simulink model "HighLevelLowLevel_SITLA 2"  (R2023b)
settings: Solver=FixedStepAuto  StartTime=0.0  StopTime=100  FixedStep=0.0025  RelTol=1e-3
InitFcn:
  | startup
model workspace (MAT data in the model file):
  Cd = 2.24197803e-06
  Ct = 0.00010297
  Ixx = 113600
  Iyy = 113600
  Izz = 22620
  h = 0.05
values from neighbouring files (symbols this model uses):
  g = 9.806    [startup.m]
  I = [0.42 0 0; 0 0.42 0; 0 0 0.642]    [startup.m]
  l = 0.053336    [startup.m]
  m = 7.4    [startup.m]
  sample_rate = 0.0025    [startup.m]
libraries: simulink_extras x12, matrix_library x9, AP_Conector0x2810x29 x2, aerolibanimutils x1, shared6dof x1, commchan3 x1
settings Model: Creator=awahm  LastModifiedBy=okmatteson
settings OptimizationCC: DefaultParameterBehavior=Inlined  UseDivisionForNetSlopeComputation=on  GainParamInheritBuiltInType=on  UseFloatMulNetSlope=on  OptimizeBlockIOStorage=off  ZeroExternalMemoryAtStartup=off  ZeroInternalMemoryAtStartup=off  LifeSpan=1  OptimizeDataStoreBuffers=off  BusAssignmentInplaceUpdate=off
settings DebuggingCC: SFUnexpectedBacktrackingDiag=warning  SFNoUnconditionalDefaultTransitionDiag=warning
settings RTWCC: GenerateReport=on  BuildConfiguration=Debug  LaunchReport=on  TargetLang=C++
settings CodeAppCC: ForceParamTrailComments=on  MATLABSourceComments=on  EnableCustomComments=on
settings GRTTargetCC: TargetLangStandard=C++11 (ISO)  CombineSignalStateStructs=on  CodeInterfacePackaging=C++ class  SupportVariableSizeSignals=on  MultiInstanceErrorCode=Warning

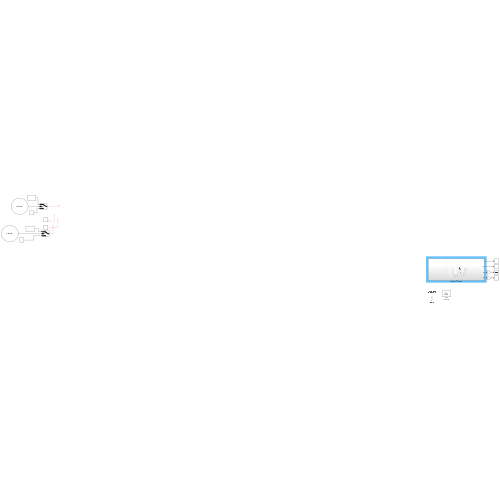
[thumbnail: Simulink's stored preview of the top-level diagram]
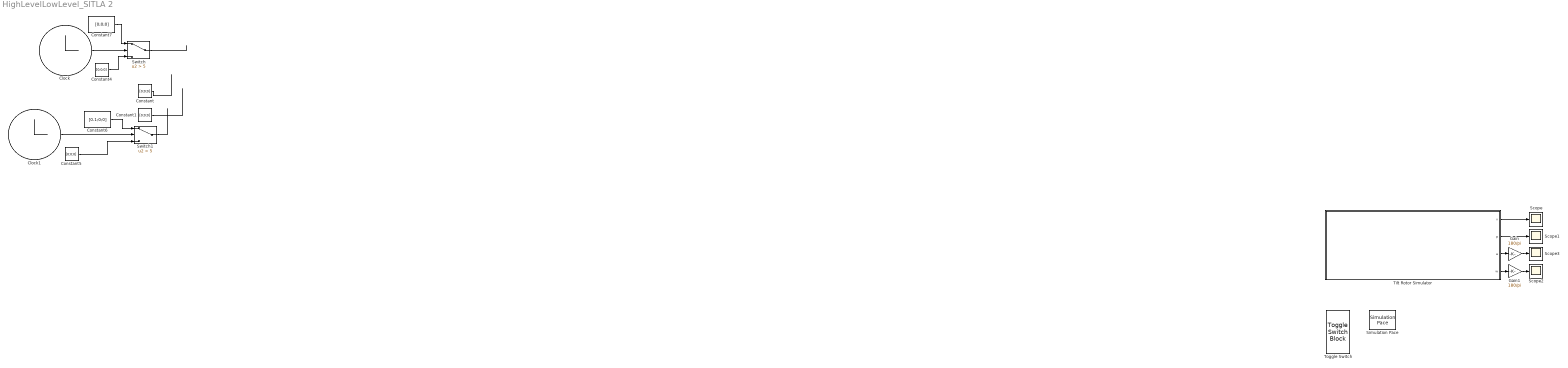
== system HighLevelLowLevel_SITLA 2 ==
  Clock : Clock
  Clock1 : Clock
  Constant{,1,4..5,7} (5 alike) : Constant  Value=[0;0;0]
  Constant6 : Constant  Value=[0.1;0;0]
  Gain : Gain  Gain=180/pi
  Gain1 : Gain  Gain=180/pi
  Scope{,1..3} (4 alike) : Scope
  Simulation Pace : aerolibanimutils/Simulation Pace  SimulationPace=1  SleepMode=Auto  OutputPaceError=off  SampleTime=sample_rate
  Switch : Switch  Criteria=u2 > Threshold  Threshold=5  SaturateOnIntegerOverflow=off  InputSameDT=off
  Switch1 : Switch  Criteria=u2 > Threshold  Threshold=5  SaturateOnIntegerOverflow=off  InputSameDT=off
  Tilt Rotor Simulator : Subsystem
  Toggle Switch : ToggleSwitchBlock
      settings: Values={{'Manual', 'Autonomous'}, [0 1]}
  wires:
  Constant/1 -> ?
  Switch1/1 -> ?
  Constant1/1 -> ?
  Clock/1 -> Switch/2
  Constant7/1 -> Switch/1
  Switch/1 -> ?
  Constant4/1 -> Switch/3
  Clock1/1 -> Switch1/2
  Constant6/1 -> Switch1/1
  Constant5/1 -> Switch1/3
  Tilt Rotor Simulator/1(v) -> Scope/1
  Tilt Rotor Simulator/4(w) -> Gain1/1
  Tilt Rotor Simulator/3(a) -> Gain/1
  Tilt Rotor Simulator/2(p) -> Scope1/1
  Gain/1 -> Scope3/1
  Gain1/1 -> Scope2/1

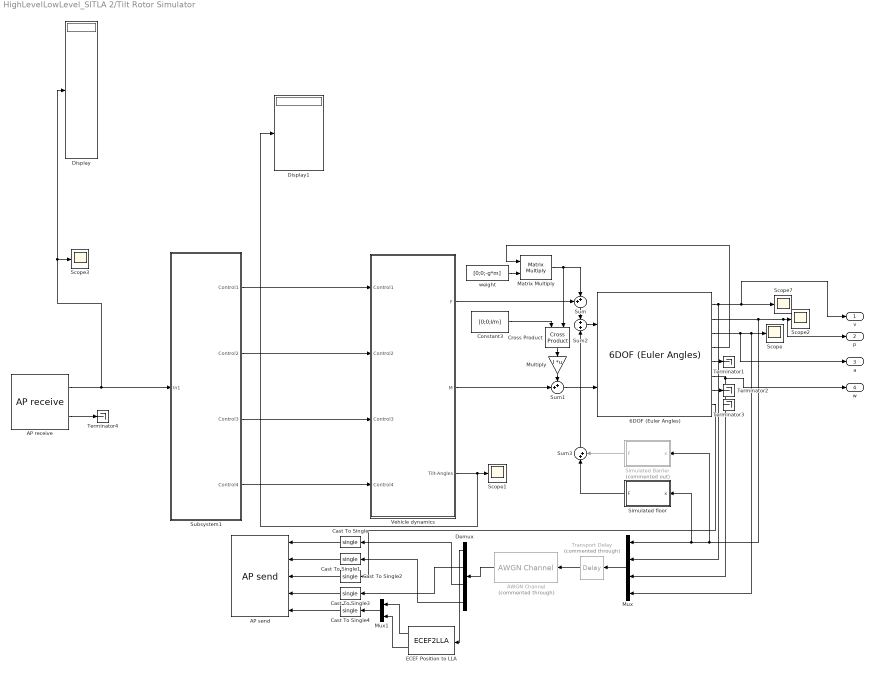
== system HighLevelLowLevel_SITLA 2/Tilt Rotor Simulator ==
  6DOF (Euler Angles) : shared6dof/6DOF (Euler Angles)  units=Metric (MKS)  mtype=Fixed  rep=Euler Angles  xme_0=[0 0 0]  Vm_0=[0 0 0]  eul_0=[0 0 0]  pm_0=[0 0 0]  mass_0=7.4  mass_e=0.5  mass_f=2.0  inertia=I  inertia_e=eye(3)  inertia_f=2*eye(3)  k_quat=1.0  vre_flag=on  abi_flag=off  aMode=0  xme_statename=''  Vm_statename=''  eul_statename=''  quat_statename=''  pm_statename=''  mass_statename=''
  AP receive : AP_Conector0x2810x29/AP receive  SystemSampleTime=-1  VariantActivationTime=update diagram  AllowFlexibleInterface=on  Latency=0  AutoFrameSizeCalculation=off
  AP send : AP_Conector0x2810x29/AP send  SystemSampleTime=-1  VariantActivationTime=update diagram  AllowFlexibleInterface=on  Latency=0  AutoFrameSizeCalculation=off
  AWGN Channel : commchan3/AWGN Channel  Commented=through  LegacyMode=on  NoiseMethod="Signal to noise ratio  (SNR)"  noiseMode="Signal to noise ratio  (SNR)"  EbNo=10  EsNo=10  SNR=10  BitsPerSymbol=1  SignalPower=1  SamplesPerSymbol=1  SymbolPeriod=1  VarianceSource=Parameter  Variance=1  RandomStream=Global stream  Seed=67  SimulateUsing=Code generation
  Cast To Single{,1..4} (5 alike) : DataTypeConversion  OutDataTypeStr=single  SaturateOnIntegerOverflow=off  RndMeth=Floor
  Constant3 : Constant  Value=[0;0;l/m]
  Cross Product : matrix_library/Cross Product
  Demux : Demux
  Display : Display
  Display1 : Display
  ECEF Position to LLA : ECEF2LLA
  Matrix Multiply : Product  Multiplication=Matrix(*)
  Multiply : Gain  Gain=I  Multiplication=Matrix(K*u)
  Mux : Mux
  Mux1 : Mux  Inputs=2
  Scope{,1..3,7} (5 alike) : Scope
  Simulated Barrier : MATLAB Function  Commented=on  TreatAsAtomicUnit=on  mask{x1=[0; -5], x2=[0; 5], E=1000000, thickness=0.1, A=0.5^2}
  Simulated floor : MATLAB Function  TreatAsAtomicUnit=on  mask{x1=[-100; -0.1], x2=[100; -0.1], E=1000000, thickness=0.1, A=0.5^2}
  Subsystem1 : Subsystem
  Sum : Sum  Inputs=++|
  Sum1 : Sum  Inputs=++|
  Sum2 : Sum  Inputs=+|+
  Sum3 : Sum  Inputs=|++
  Terminator{1..4} (4 alike) : Terminator
  Transport Delay : TransportDelay  Commented=through  DelayTime=0.006
  Vehicle dynamics : Subsystem
  weight : Constant  Value=[0;0;-g*m]
  v : Outport
  p : Outport  Port=2
  a : Outport  Port=3
  w : Outport  Port=4
  wires:
  6DOF (Euler Angles)/2 -> p/1, Scope2/1, Simulated Barrier/1(x), Simulated floor/1(x), Mux/1
  Mux/1 -> Transport Delay/1
  6DOF (Euler Angles)/6 -> w/1, Mux/3
  weight/1 -> Matrix Multiply/2
  Matrix Multiply/1 -> Cross Product/2, Sum/2
  Vehicle dynamics/1(F) -> Sum/1
  6DOF (Euler Angles)/8 -> Cast To Single2/1
  Vehicle dynamics/3(Tilt-Angles) -> Display1/1, Scope1/1
  Sum1/1 -> 6DOF (Euler Angles)/2
  AWGN Channel/1 -> Demux/1
  6DOF (Euler Angles)/1 -> v/1, Scope7/1, Mux/2
  Cross Product/1 -> Multiply/1
  Vehicle dynamics/2(M) -> Sum1/2
  6DOF (Euler Angles)/3 -> a/1, Mux/4, Scope/1
  6DOF (Euler Angles)/7 -> Terminator2/1
  Transport Delay/1 -> AWGN Channel/1
  6DOF (Euler Angles)/4 -> Matrix Multiply/1
  Constant3/1 -> Cross Product/1
  Multiply/1 -> Sum1/1
  6DOF (Euler Angles)/5 -> Terminator1/1
  Sum/1 -> Sum2/1
  Sum2/1 -> 6DOF (Euler Angles)/1
  Simulated Barrier/1(F) -> Sum3/2
  AP receive/2 -> Terminator4/1
  AP receive/1 -> Scope3/1, Display/1, Subsystem1/1(In1)
  Demux/1 -> ECEF Position to LLA/1
  Demux/2 -> Cast To Single3/1
  Demux/4 -> Cast To Single1/1
  Demux/3 -> Cast To Single/1
  Cast To Single/1 -> AP send/1
  Cast To Single1/1 -> AP send/2
  Cast To Single4/1 -> AP send/5
  Subsystem1/1(Control1) -> Vehicle dynamics/1(Control1)
  Subsystem1/2(Control2) -> Vehicle dynamics/2(Control2)
  Subsystem1/3(Control3) -> Vehicle dynamics/3(Control3)
  Subsystem1/4(Control4) -> Vehicle dynamics/4(Control4)
  ECEF Position to LLA/1 -> Mux1/1
  ECEF Position to LLA/2 -> Mux1/2
  Mux1/1 -> Cast To Single4/1
  Cast To Single3/1 -> AP send/4
  Cast To Single2/1 -> AP send/3
  Simulated floor/1(F) -> Sum3/1
  Sum3/1 -> Sum2/2

== system HighLevelLowLevel_SITLA 2/Tilt Rotor Simulator/Subsystem1 ==
  In1 : Inport
  Demux1 : Demux  Outputs=16
  Mux{,1..3} (4 alike) : Mux  Inputs=3
  Scope : Scope
  Scope1 : Scope
  Subsystem : Subsystem
  Control1 : Outport
  Control2 : Outport  Port=2
  Control3 : Outport  Port=3
  Control4 : Outport  Port=4
  wires:
  Demux1/1 -> Subsystem/1(In1)
  Demux1/2 -> Subsystem/2(In2)
  Demux1/3 -> Subsystem/3(In3)
  Demux1/4 -> Subsystem/4(In4)
  Demux1/5 -> Scope1/1, Subsystem/5(In5)
  Demux1/6 -> Subsystem/6(In6)
  Demux1/8 -> Subsystem/8(In8)
  Demux1/7 -> Subsystem/7(In7)
  Demux1/9 -> Subsystem/9(In9)
  Demux1/10 -> Subsystem/10(In10)
  Demux1/11 -> Subsystem/11(In11)
  Demux1/12 -> Subsystem/12(In12)
  In1/1 -> Demux1/1
  Subsystem/1(Out1) -> Mux/3
  Subsystem/5(Out5) -> Mux/2, Scope/1
  Subsystem/9(Out9) -> Mux/1
  Mux/1 -> Control1/1
  Mux1/1 -> Control2/1
  Subsystem/2(Out2) -> Mux1/3
  Subsystem/6(Out6) -> Mux1/2
  Subsystem/10(Out10) -> Mux1/1
  Mux2/1 -> Control3/1
  Subsystem/7(Out7) -> Mux2/2
  Subsystem/3(Out3) -> Mux2/3
  Subsystem/11(Out11) -> Mux2/1
  Mux3/1 -> Control4/1
  Subsystem/4(Out4) -> Mux3/3
  Subsystem/8(Out8) -> Mux3/2
  Subsystem/12(Out12) -> Mux3/1

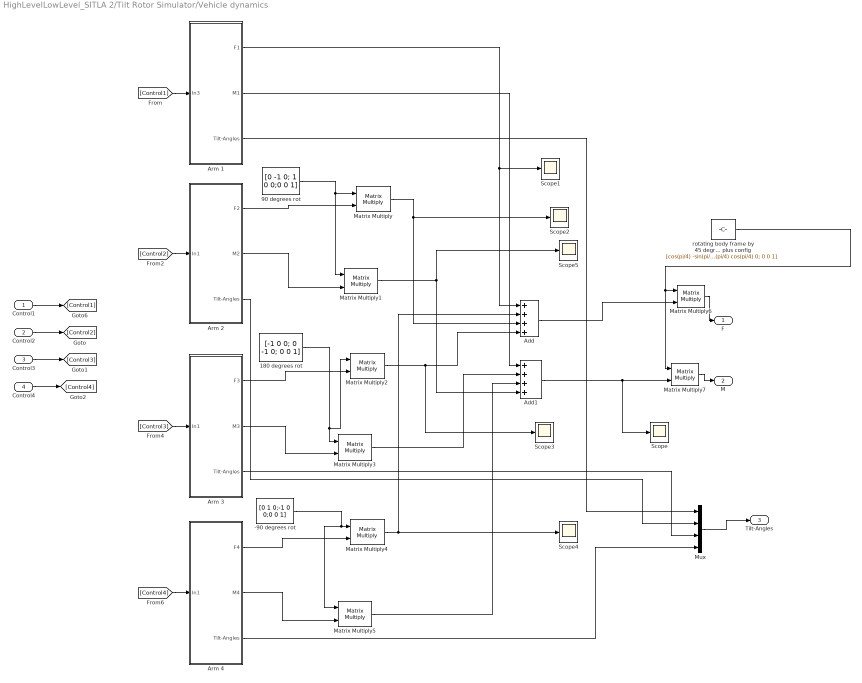
== system HighLevelLowLevel_SITLA 2/Tilt Rotor Simulator/Vehicle dynamics ==
  Control1 : Inport
  Control2 : Inport  Port=2
  Control3 : Inport  Port=3
  Control4 : Inport  Port=4
  -90 degrees rot : Constant  Value=[0 1 0;-1 0 0;0 0 1]
  180 degrees rot : Constant  Value=[-1 0 0; 0 -1 0; 0 0 1]
  90 degrees rot : Constant  Value=[0 -1 0; 1 0 0;0 0 1]
  Add : Sum  Inputs=++++
  Add1 : Sum  Inputs=++++
  Arm 1 : Subsystem
  Arm 2 : Subsystem
  Arm 3 : Subsystem
  Arm 4 : Subsystem
  Matrix Multiply{,1..7} (8 alike) : Product  Multiplication=Matrix(*)
  Mux : Mux
  Scope{,1..5} (6 alike) : Scope
  rotating body frame by 45 degrees to X config because vehicle dynamics was done in plus config : Constant  Value=|
      | [cos(pi/4) -sin(pi/4) 0;
      | sin(pi/4) cos(pi/4) 0;
      | 0 0 1]
  F : Outport
  M : Outport  Port=2
  Tilt-Angles : Outport  Port=3
  wires:
  Control1/1 -> [Control1]
  Control2/1 -> [Control2]
  Control3/1 -> [Control3]
  Control4/1 -> [Control4]
  [Control1] -> Arm 1/1(In3)
  Arm 1/1(F1) -> Add/1, Scope1/1
  Arm 1/2(M1) -> Add1/1
  90 degrees rot/1 -> Matrix Multiply1/1, Matrix Multiply/1
  Arm 2/1(F2) -> Matrix Multiply/2
  Matrix Multiply/1 -> Scope2/1, Add/3
  Arm 2/2(M2) -> Matrix Multiply1/2
  Matrix Multiply1/1 -> Add1/4, Scope5/1
  [Control2] -> Arm 2/1(In1)
  -90 degrees rot/1 -> Matrix Multiply5/1, Matrix Multiply4/1
  Arm 3/1(F3) -> Matrix Multiply2/2
  Matrix Multiply3/1 -> Add1/2
  [Control3] -> Arm 3/1(In1)
  Arm 3/2(M3) -> Matrix Multiply3/2
  180 degrees rot/1 -> Matrix Multiply3/1, Matrix Multiply2/1
  Arm 4/2(M4) -> Matrix Multiply5/2
  Arm 4/1(F4) -> Matrix Multiply4/2
  Matrix Multiply5/1 -> Add1/3
  [Control4] -> Arm 4/1(In1)
  Matrix Multiply2/1 -> Scope3/1, Add/4
  Matrix Multiply4/1 -> Add/2, Scope4/1
  rotating body frame by 45 degrees to X config because vehicle dynamics was done in plus config/1 -> Matrix Multiply6/1, Matrix Multiply7/1
  Add/1 -> Matrix Multiply6/2
  Add1/1 -> Matrix Multiply7/2, Scope/1
  Matrix Multiply7/1 -> M/1
  Matrix Multiply6/1 -> F/1
  Arm 1/3(Tilt-Angles) -> Mux/1
  Arm 2/3(Tilt-Angles) -> Mux/2
  Arm 3/3(Tilt-Angles) -> Mux/3
  Arm 4/3(Tilt-Angles) -> Mux/4
  Mux/1 -> Tilt-Angles/1

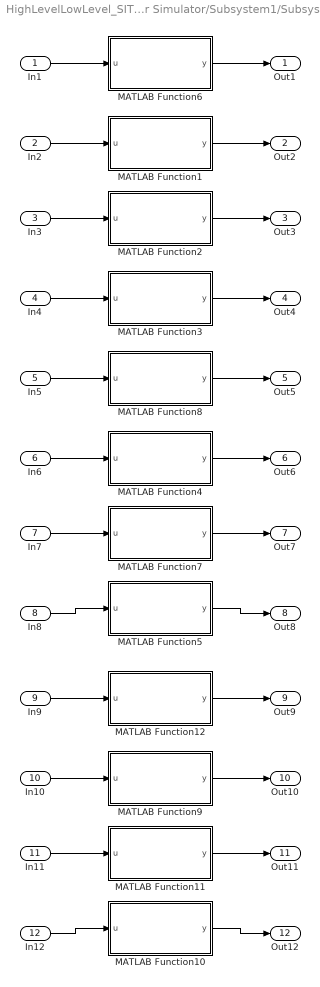
== system HighLevelLowLevel_SITLA 2/Tilt Rotor Simulator/Subsystem1/Subsystem ==
  In1 : Inport
  In2 : Inport  Port=2
  In3 : Inport  Port=3
  In4 : Inport  Port=4
  In5 : Inport  Port=5
  In6 : Inport  Port=6
  In7 : Inport  Port=7
  In8 : Inport  Port=8
  In9 : Inport  Port=9
  In10 : Inport  Port=10
  In11 : Inport  Port=11
  In12 : Inport  Port=12
  MATLAB Function1 : MATLAB Function  TreatAsAtomicUnit=on  mask{min_in=1000, min_out=0, max_in=2000, max_out=633}
  MATLAB Function10 : MATLAB Function  TreatAsAtomicUnit=on  mask{min_in=682, min_out=-1.57, max_in=2318, max_out=1.57}
  MATLAB Function11 : MATLAB Function  TreatAsAtomicUnit=on  mask{min_in=682, min_out=-1.57, max_in=2318, max_out=1.57}
  MATLAB Function12 : MATLAB Function  TreatAsAtomicUnit=on  mask{min_in=682, min_out=-1.57, max_in=2318, max_out=1.57}
  MATLAB Function2 : MATLAB Function  TreatAsAtomicUnit=on  mask{min_in=1000, min_out=0, max_in=2000, max_out=633}
  MATLAB Function3 : MATLAB Function  TreatAsAtomicUnit=on  mask{min_in=1000, min_out=0, max_in=2000, max_out=633}
  MATLAB Function4 : MATLAB Function  TreatAsAtomicUnit=on  mask{min_in=682, min_out=-1.57, max_in=2318, max_out=1.57}
  MATLAB Function5 : MATLAB Function  TreatAsAtomicUnit=on  mask{min_in=682, min_out=-1.57, max_in=2318, max_out=1.57}
  MATLAB Function6 : MATLAB Function  TreatAsAtomicUnit=on  mask{min_in=1000, min_out=0, max_in=2000, max_out=633}
  MATLAB Function7 : MATLAB Function  TreatAsAtomicUnit=on  mask{min_in=682, min_out=-1.57, max_in=2318, max_out=1.57}
  MATLAB Function8 : MATLAB Function  TreatAsAtomicUnit=on  mask{min_in=682, min_out=-1.57, max_in=2318, max_out=1.57}
  MATLAB Function9 : MATLAB Function  TreatAsAtomicUnit=on  mask{min_in=682, min_out=-1.57, max_in=2318, max_out=1.57}
  Out1 : Outport
  Out2 : Outport  Port=2
  Out3 : Outport  Port=3
  Out4 : Outport  Port=4
  Out5 : Outport  Port=5
  Out6 : Outport  Port=6
  Out7 : Outport  Port=7
  Out8 : Outport  Port=8
  Out9 : Outport  Port=9
  Out10 : Outport  Port=10
  Out11 : Outport  Port=11
  Out12 : Outport  Port=12
  wires:
  In1/1 -> MATLAB Function6/1(u)
  MATLAB Function6/1(y) -> Out1/1
  In2/1 -> MATLAB Function1/1(u)
  MATLAB Function1/1(y) -> Out2/1
  MATLAB Function2/1(y) -> Out3/1
  In3/1 -> MATLAB Function2/1(u)
  In4/1 -> MATLAB Function3/1(u)
  MATLAB Function3/1(y) -> Out4/1
  In5/1 -> MATLAB Function8/1(u)
  MATLAB Function8/1(y) -> Out5/1
  MATLAB Function4/1(y) -> Out6/1
  In6/1 -> MATLAB Function4/1(u)
  In7/1 -> MATLAB Function7/1(u)
  MATLAB Function7/1(y) -> Out7/1
  In8/1 -> MATLAB Function5/1(u)
  MATLAB Function5/1(y) -> Out8/1
  In9/1 -> MATLAB Function12/1(u)
  MATLAB Function12/1(y) -> Out9/1
  MATLAB Function9/1(y) -> Out10/1
  In10/1 -> MATLAB Function9/1(u)
  In11/1 -> MATLAB Function11/1(u)
  MATLAB Function11/1(y) -> Out11/1
  In12/1 -> MATLAB Function10/1(u)
  MATLAB Function10/1(y) -> Out12/1

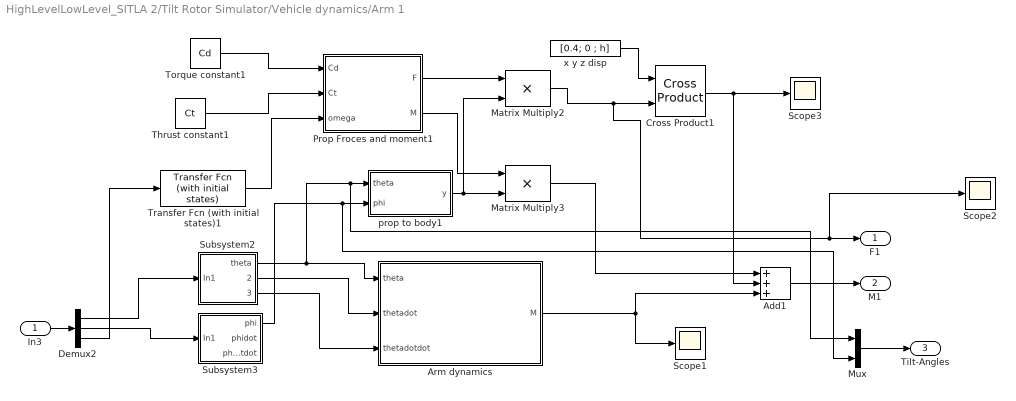
== system HighLevelLowLevel_SITLA 2/Tilt Rotor Simulator/Vehicle dynamics/Arm 1 ==
  In3 : Inport
  Add1 : Sum  Inputs=+++
  Arm dynamics : Subsystem
  Cross Product1 : matrix_library/Cross Product
  Demux2 : Demux  Outputs=3
  Matrix Multiply2 : Product
  Matrix Multiply3 : Product
  Mux : Mux  Inputs=2
  Prop Froces and moment1 : Subsystem
  Scope1 : Scope
  Scope2 : Scope
  Scope3 : Scope
  Subsystem2 : Subsystem
  Subsystem3 : Subsystem
  Thrust constant1 : Constant  Value=Ct
  Torque constant1 : Constant  Value=Cd
  Transfer Fcn (with initial states)1 : simulink_extras/Additional Linear/Transfer Fcn (with initial states)  N=[153.35]  D=[1 20.06 153.35]  X0=0
  prop to body1 : MATLAB Function  TreatAsAtomicUnit=on
  x y z disp : Constant  Value=[0.4; 0 ; h]
  F1 : Outport
  M1 : Outport  Port=2
  Tilt-Angles : Outport  Port=3
  wires:
  x y z disp/1 -> Cross Product1/1
  Subsystem2/2(thetadot) -> Arm dynamics/2(thetadot)
  Cross Product1/1 -> Add1/2, Scope3/1
  In3/1 -> Demux2/1
  Prop Froces and moment1/1(F) -> Matrix Multiply2/1
  Arm dynamics/1(M) -> Add1/3, Scope1/1
  Demux2/2 -> Subsystem3/1(In1)
  Thrust constant1/1 -> Prop Froces and moment1/2(Ct)
  Torque constant1/1 -> Prop Froces and moment1/1(Cd)
  Add1/1 -> M1/1
  Matrix Multiply3/1 -> Add1/1
  prop to body1/1(y) -> Matrix Multiply3/2, Matrix Multiply2/2
  Prop Froces and moment1/2(M) -> Matrix Multiply3/1
  Demux2/1 -> Subsystem2/1(In1)
  Subsystem2/1(theta) -> Arm dynamics/1(theta), Mux/1, prop to body1/1(theta)
  Matrix Multiply2/1 -> Cross Product1/2, Scope2/1, F1/1
  Subsystem3/1(phi) -> Mux/2, prop to body1/2(phi)
  Subsystem2/3(thetadotdot) -> Arm dynamics/3(thetadotdot)
  Demux2/3 -> Transfer Fcn (with initial states)1/1
  Transfer Fcn (with initial states)1/1 -> Prop Froces and moment1/3(omega)
  Mux/1 -> Tilt-Angles/1

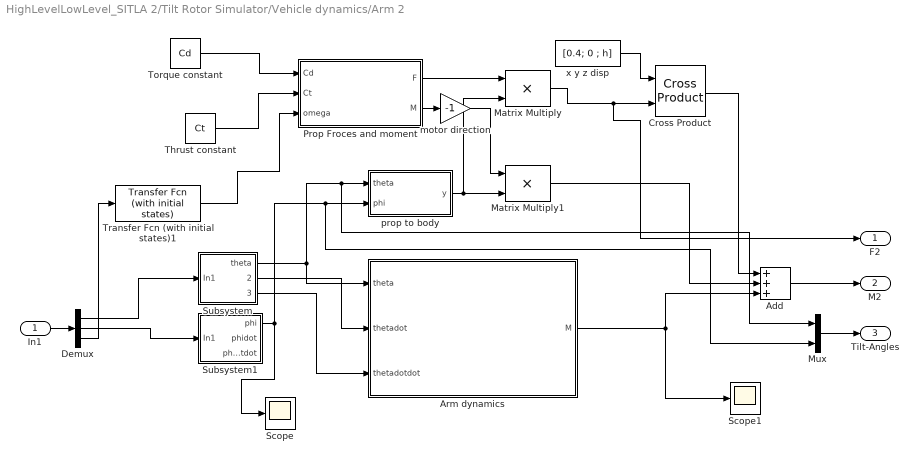
== system HighLevelLowLevel_SITLA 2/Tilt Rotor Simulator/Vehicle dynamics/Arm 2 ==
  In1 : Inport
  Add : Sum  Inputs=+++
  Arm dynamics : Subsystem
  Cross Product : matrix_library/Cross Product
  Demux : Demux  Outputs=3
  Matrix Multiply : Product
  Matrix Multiply1 : Product
  Mux : Mux  Inputs=2
  Prop Froces and moment : Subsystem
  Scope : Scope
  Scope1 : Scope
  Subsystem : Subsystem
  Subsystem1 : Subsystem
  Thrust constant : Constant  Value=Ct
  Torque constant : Constant  Value=Cd
  Transfer Fcn (with initial states)1 : simulink_extras/Additional Linear/Transfer Fcn (with initial states)  N=[153.35]  D=[1 20.06 153.35]  X0=0
  motor direction : Gain  Gain=-1
  prop to body : MATLAB Function  TreatAsAtomicUnit=on
  x y z disp : Constant  Value=[0.4; 0 ; h]
  F2 : Outport
  M2 : Outport  Port=2
  Tilt-Angles : Outport  Port=3
  wires:
  prop to body/1(y) -> Matrix Multiply1/2, Matrix Multiply/2
  Demux/2 -> Subsystem1/1(In1)
  Matrix Multiply/1 -> Cross Product/2, F2/1
  Prop Froces and moment/1(F) -> Matrix Multiply/1
  Subsystem/1(theta) -> Arm dynamics/1(theta), Mux/1, prop to body/1(theta)
  Matrix Multiply1/1 -> Add/2
  Prop Froces and moment/2(M) -> motor direction/1
  Subsystem1/1(phi) -> Scope/1, Mux/2, prop to body/2(phi)
  Demux/1 -> Subsystem/1(In1)
  x y z disp/1 -> Cross Product/1
  Add/1 -> M2/1
  Torque constant/1 -> Prop Froces and moment/1(Cd)
  Thrust constant/1 -> Prop Froces and moment/2(Ct)
  Cross Product/1 -> Add/1
  In1/1 -> Demux/1
  Subsystem/2(thetadot) -> Arm dynamics/2(thetadot)
  Subsystem/3(thetadotdot) -> Arm dynamics/3(thetadotdot)
  Arm dynamics/1(M) -> Add/3, Scope1/1
  Demux/3 -> Transfer Fcn (with initial states)1/1
  motor direction/1 -> Matrix Multiply1/1
  Transfer Fcn (with initial states)1/1 -> Prop Froces and moment/3(omega)
  Mux/1 -> Tilt-Angles/1

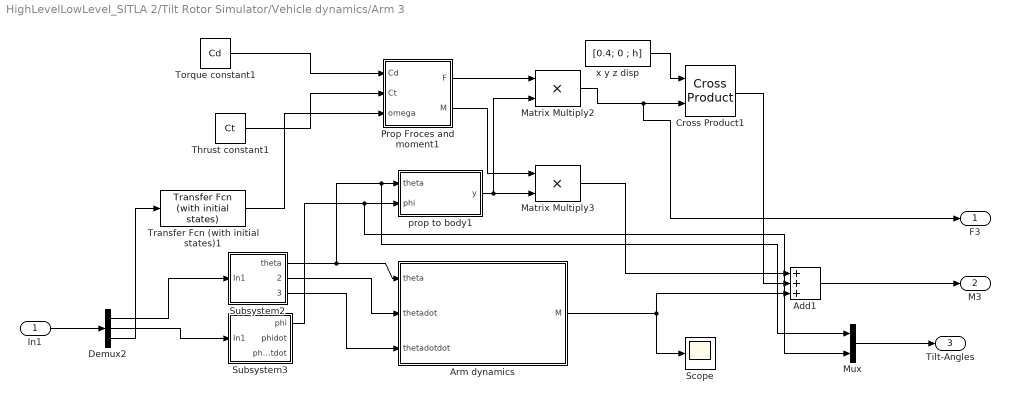
== system HighLevelLowLevel_SITLA 2/Tilt Rotor Simulator/Vehicle dynamics/Arm 3 ==
  In1 : Inport
  Add1 : Sum  Inputs=+++
  Arm dynamics : Subsystem
  Cross Product1 : matrix_library/Cross Product
  Demux2 : Demux  Outputs=3
  Matrix Multiply2 : Product
  Matrix Multiply3 : Product
  Mux : Mux  Inputs=2
  Prop Froces and moment1 : Subsystem
  Scope : Scope
  Subsystem2 : Subsystem
  Subsystem3 : Subsystem
  Thrust constant1 : Constant  Value=Ct
  Torque constant1 : Constant  Value=Cd
  Transfer Fcn (with initial states)1 : simulink_extras/Additional Linear/Transfer Fcn (with initial states)  N=[153.35]  D=[1 20.06 153.35]  X0=0
  prop to body1 : MATLAB Function  TreatAsAtomicUnit=on
  x y z disp : Constant  Value=[0.4; 0 ; h]
  F3 : Outport
  M3 : Outport  Port=2
  Tilt-Angles : Outport  Port=3
  wires:
  x y z disp/1 -> Cross Product1/1
  Subsystem2/2(thetadot) -> Arm dynamics/2(thetadot)
  Cross Product1/1 -> Add1/2
  In1/1 -> Demux2/1
  Prop Froces and moment1/1(F) -> Matrix Multiply2/1
  Arm dynamics/1(M) -> Add1/3, Scope/1
  Demux2/2 -> Subsystem3/1(In1)
  Thrust constant1/1 -> Prop Froces and moment1/2(Ct)
  Torque constant1/1 -> Prop Froces and moment1/1(Cd)
  Add1/1 -> M3/1
  Matrix Multiply3/1 -> Add1/1
  prop to body1/1(y) -> Matrix Multiply3/2, Matrix Multiply2/2
  Prop Froces and moment1/2(M) -> Matrix Multiply3/1
  Demux2/1 -> Subsystem2/1(In1)
  Subsystem2/1(theta) -> Arm dynamics/1(theta), Mux/1, prop to body1/1(theta)
  Demux2/3 -> Transfer Fcn (with initial states)1/1
  Matrix Multiply2/1 -> Cross Product1/2, F3/1
  Subsystem3/1(phi) -> Mux/2, prop to body1/2(phi)
  Subsystem2/3(thetadotdot) -> Arm dynamics/3(thetadotdot)
  Transfer Fcn (with initial states)1/1 -> Prop Froces and moment1/3(omega)
  Mux/1 -> Tilt-Angles/1

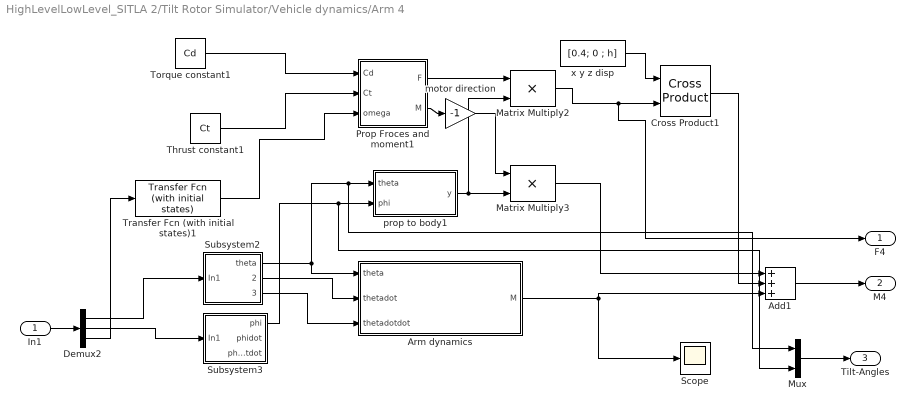
== system HighLevelLowLevel_SITLA 2/Tilt Rotor Simulator/Vehicle dynamics/Arm 4 ==
  In1 : Inport
  Add1 : Sum  Inputs=+++
  Arm dynamics : Subsystem
  Cross Product1 : matrix_library/Cross Product
  Demux2 : Demux  Outputs=3
  Matrix Multiply2 : Product
  Matrix Multiply3 : Product
  Mux : Mux  Inputs=2
  Prop Froces and moment1 : Subsystem
  Scope : Scope
  Subsystem2 : Subsystem
  Subsystem3 : Subsystem
  Thrust constant1 : Constant  Value=Ct
  Torque constant1 : Constant  Value=Cd
  Transfer Fcn (with initial states)1 : simulink_extras/Additional Linear/Transfer Fcn (with initial states)  N=[153.35]  D=[1 20.06 153.35]  X0=0
  motor direction : Gain  Gain=-1
  prop to body1 : MATLAB Function  TreatAsAtomicUnit=on
  x y z disp : Constant  Value=[0.4; 0 ; h]
  F4 : Outport
  M4 : Outport  Port=2
  Tilt-Angles : Outport  Port=3
  wires:
  x y z disp/1 -> Cross Product1/1
  Subsystem2/2(thetadot) -> Arm dynamics/2(thetadot)
  Cross Product1/1 -> Add1/2
  In1/1 -> Demux2/1
  Prop Froces and moment1/1(F) -> Matrix Multiply2/1
  Arm dynamics/1(M) -> Add1/3, Scope/1
  Demux2/2 -> Subsystem3/1(In1)
  Thrust constant1/1 -> Prop Froces and moment1/2(Ct)
  Torque constant1/1 -> Prop Froces and moment1/1(Cd)
  Add1/1 -> M4/1
  Matrix Multiply3/1 -> Add1/1
  prop to body1/1(y) -> Matrix Multiply3/2, Matrix Multiply2/2
  Prop Froces and moment1/2(M) -> motor direction/1
  Demux2/1 -> Subsystem2/1(In1)
  Subsystem2/1(theta) -> Arm dynamics/1(theta), Mux/1, prop to body1/1(theta)
  Matrix Multiply2/1 -> Cross Product1/2, F4/1
  Subsystem3/1(phi) -> Mux/2, prop to body1/2(phi)
  Subsystem2/3(thetadotdot) -> Arm dynamics/3(thetadotdot)
  Demux2/3 -> Transfer Fcn (with initial states)1/1
  motor direction/1 -> Matrix Multiply3/1
  Transfer Fcn (with initial states)1/1 -> Prop Froces and moment1/3(omega)
  Mux/1 -> Tilt-Angles/1

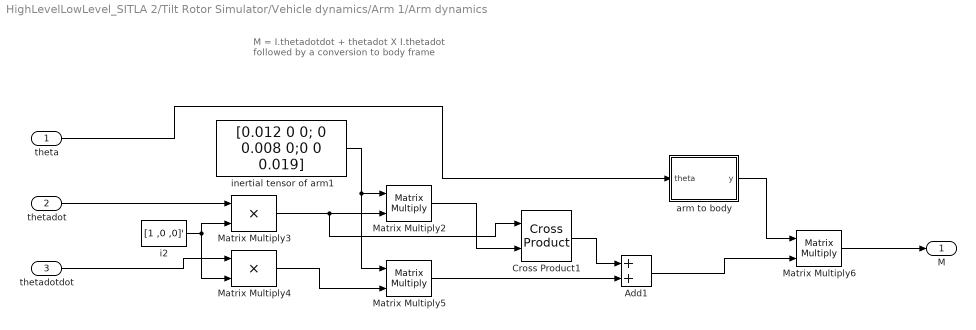
== system HighLevelLowLevel_SITLA 2/Tilt Rotor Simulator/Vehicle dynamics/Arm 1/Arm dynamics ==
  note: M = I.thetadotdot + thetadot X I.thetadot
      | followed by a conversion to body frame
  theta : Inport
  thetadot : Inport  Port=2
  thetadotdot : Inport  Port=3
  Add1 : Sum
  Cross Product1 : matrix_library/Cross Product
  Matrix Multiply2 : Product  Multiplication=Matrix(*)
  Matrix Multiply3 : Product
  Matrix Multiply4 : Product
  Matrix Multiply5 : Product  Multiplication=Matrix(*)
  Matrix Multiply6 : Product  Multiplication=Matrix(*)
  arm to body : MATLAB Function  TreatAsAtomicUnit=on
  i2 : Constant  Value=[1 ,0 ,0]'
  inertial tensor of arm1 : Constant  Value=[0.012 0 0; 0 0.008 0;0 0 0.019]
  M : Outport
  wires:
  Matrix Multiply3/1 -> Cross Product1/1, Matrix Multiply2/2
  inertial tensor of arm1/1 -> Matrix Multiply5/1, Matrix Multiply2/1
  thetadotdot/1 -> Matrix Multiply4/1
  Matrix Multiply4/1 -> Matrix Multiply5/2
  Matrix Multiply5/1 -> Add1/2
  i2/1 -> Matrix Multiply4/2, Matrix Multiply3/2
  arm to body/1(y) -> Matrix Multiply6/1
  Matrix Multiply2/1 -> Cross Product1/2
  Cross Product1/1 -> Add1/1
  Add1/1 -> Matrix Multiply6/2
  thetadot/1 -> Matrix Multiply3/1
  Matrix Multiply6/1 -> M/1
  theta/1 -> arm to body/1(theta)

== system HighLevelLowLevel_SITLA 2/Tilt Rotor Simulator/Vehicle dynamics/Arm 1/Prop Froces and moment1 ==
  note: T = Ctx w^2
      | Q = Cd x w^2
  Cd : Inport
  Ct : Inport  Port=2
  omega : Inport  Port=3
  Product{,1..3} (4 alike) : Product
  F : Outport
  M : Outport  Port=2
  wires:
  omega/1 -> Product3/1, Product2/2, Product1/2, Product/2
  Ct/1 -> Product2/1
  Product2/1 -> Product3/2
  Product3/1 -> F/1
  Product/1 -> Product1/1
  Product1/1 -> M/1
  Cd/1 -> Product/1

== system HighLevelLowLevel_SITLA 2/Tilt Rotor Simulator/Vehicle dynamics/Arm 1/Subsystem2 ==
  In1 : Inport
  Derivative : Derivative
  Derivative1 : Derivative  CoefficientInTFapproximation=1
  Scope : Scope
  Scope1 : Scope
  Scope2 : Scope
  Transfer Fcn (with initial states)1 : simulink_extras/Additional Linear/Transfer Fcn (with initial states)  N=[153.5000]  D="[1  20.06  153.3]"  X0=0
  theta : Outport
  thetadot : Outport  Port=2
  thetadotdot : Outport  Port=3
  wires:
  Derivative/1 -> Scope2/1, thetadot/1, Derivative1/1
  Transfer Fcn (with initial states)1/1 -> Derivative/1, Scope/1, theta/1
  Derivative1/1 -> Scope1/1, thetadotdot/1
  In1/1 -> Transfer Fcn (with initial states)1/1

== system HighLevelLowLevel_SITLA 2/Tilt Rotor Simulator/Vehicle dynamics/Arm 1/Subsystem3 ==
  In1 : Inport
  Derivative2 : Derivative
  Derivative3 : Derivative
  Scope : Scope
  Transfer Fcn (with initial states) : simulink_extras/Additional Linear/Transfer Fcn (with initial states)  N=[153.5000]  D="[1  20.06  153.3]"  X0=0
  phi : Outport
  phidot : Outport  Port=2
  phidotdot : Outport  Port=3
  wires:
  Derivative2/1 -> phidot/1, Derivative3/1
  Transfer Fcn (with initial states)/1 -> Derivative2/1, Scope/1, phi/1
  Derivative3/1 -> phidotdot/1
  In1/1 -> Transfer Fcn (with initial states)/1

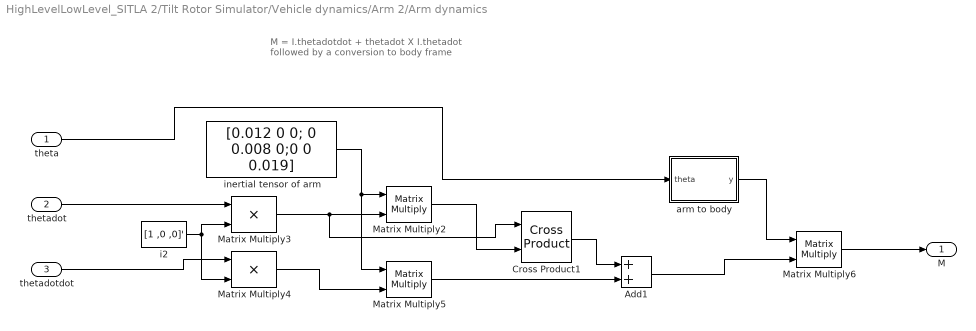
== system HighLevelLowLevel_SITLA 2/Tilt Rotor Simulator/Vehicle dynamics/Arm 2/Arm dynamics ==
  note: M = I.thetadotdot + thetadot X I.thetadot
      | followed by a conversion to body frame
  theta : Inport
  thetadot : Inport  Port=2
  thetadotdot : Inport  Port=3
  Add1 : Sum
  Cross Product1 : matrix_library/Cross Product
  Matrix Multiply2 : Product  Multiplication=Matrix(*)
  Matrix Multiply3 : Product
  Matrix Multiply4 : Product
  Matrix Multiply5 : Product  Multiplication=Matrix(*)
  Matrix Multiply6 : Product  Multiplication=Matrix(*)
  arm to body : MATLAB Function  TreatAsAtomicUnit=on
  i2 : Constant  Value=[1 ,0 ,0]'
  inertial tensor of arm : Constant  Value=[0.012 0 0; 0 0.008 0;0 0 0.019]
  M : Outport
  wires:
  Matrix Multiply3/1 -> Cross Product1/1, Matrix Multiply2/2
  inertial tensor of arm/1 -> Matrix Multiply5/1, Matrix Multiply2/1
  thetadotdot/1 -> Matrix Multiply4/1
  Matrix Multiply4/1 -> Matrix Multiply5/2
  Matrix Multiply5/1 -> Add1/2
  i2/1 -> Matrix Multiply4/2, Matrix Multiply3/2
  arm to body/1(y) -> Matrix Multiply6/1
  Matrix Multiply2/1 -> Cross Product1/2
  Cross Product1/1 -> Add1/1
  Add1/1 -> Matrix Multiply6/2
  thetadot/1 -> Matrix Multiply3/1
  Matrix Multiply6/1 -> M/1
  theta/1 -> arm to body/1(theta)

== system HighLevelLowLevel_SITLA 2/Tilt Rotor Simulator/Vehicle dynamics/Arm 2/Prop Froces and moment ==
  note: T = Ctx w^2
      | Q = Cd x w^2
  Cd : Inport
  Ct : Inport  Port=2
  omega : Inport  Port=3
  Product{,1..3} (4 alike) : Product
  F : Outport
  M : Outport  Port=2
  wires:
  omega/1 -> Product3/1, Product2/2, Product1/2, Product/2
  Ct/1 -> Product2/1
  Product2/1 -> Product3/2
  Product3/1 -> F/1
  Product/1 -> Product1/1
  Product1/1 -> M/1
  Cd/1 -> Product/1

== system HighLevelLowLevel_SITLA 2/Tilt Rotor Simulator/Vehicle dynamics/Arm 2/Subsystem ==
  In1 : Inport
  Derivative : Derivative
  Derivative1 : Derivative
  Scope : Scope
  Transfer Fcn (with initial states)1 : simulink_extras/Additional Linear/Transfer Fcn (with initial states)  N=[153.5000]  D="[1  20.06  153.3]"  X0=0
  theta : Outport
  thetadot : Outport  Port=2
  thetadotdot : Outport  Port=3
  wires:
  Derivative/1 -> thetadot/1, Derivative1/1
  Transfer Fcn (with initial states)1/1 -> Derivative/1, Scope/1, theta/1
  Derivative1/1 -> thetadotdot/1
  In1/1 -> Transfer Fcn (with initial states)1/1

== system HighLevelLowLevel_SITLA 2/Tilt Rotor Simulator/Vehicle dynamics/Arm 2/Subsystem1 ==
  In1 : Inport
  Derivative2 : Derivative
  Derivative3 : Derivative
  Scope : Scope
  Transfer Fcn (with initial states) : simulink_extras/Additional Linear/Transfer Fcn (with initial states)  N=[153.5000]  D="[1  20.06  153.3]"  X0=0
  phi : Outport
  phidot : Outport  Port=2
  phidotdot : Outport  Port=3
  wires:
  Derivative2/1 -> phidot/1, Derivative3/1
  Transfer Fcn (with initial states)/1 -> Derivative2/1, Scope/1, phi/1
  Derivative3/1 -> phidotdot/1
  In1/1 -> Transfer Fcn (with initial states)/1

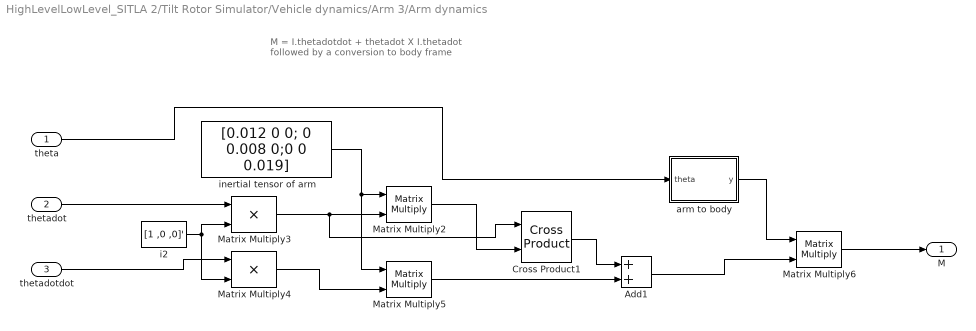
== system HighLevelLowLevel_SITLA 2/Tilt Rotor Simulator/Vehicle dynamics/Arm 3/Arm dynamics ==
  note: M = I.thetadotdot + thetadot X I.thetadot
      | followed by a conversion to body frame
  theta : Inport
  thetadot : Inport  Port=2
  thetadotdot : Inport  Port=3
  Add1 : Sum
  Cross Product1 : matrix_library/Cross Product
  Matrix Multiply2 : Product  Multiplication=Matrix(*)
  Matrix Multiply3 : Product
  Matrix Multiply4 : Product
  Matrix Multiply5 : Product  Multiplication=Matrix(*)
  Matrix Multiply6 : Product  Multiplication=Matrix(*)
  arm to body : MATLAB Function  TreatAsAtomicUnit=on
  i2 : Constant  Value=[1 ,0 ,0]'
  inertial tensor of arm : Constant  Value=[0.012 0 0; 0 0.008 0;0 0 0.019]
  M : Outport
  wires:
  Matrix Multiply3/1 -> Cross Product1/1, Matrix Multiply2/2
  inertial tensor of arm/1 -> Matrix Multiply5/1, Matrix Multiply2/1
  thetadotdot/1 -> Matrix Multiply4/1
  Matrix Multiply4/1 -> Matrix Multiply5/2
  Matrix Multiply5/1 -> Add1/2
  i2/1 -> Matrix Multiply4/2, Matrix Multiply3/2
  arm to body/1(y) -> Matrix Multiply6/1
  Matrix Multiply2/1 -> Cross Product1/2
  Cross Product1/1 -> Add1/1
  Add1/1 -> Matrix Multiply6/2
  thetadot/1 -> Matrix Multiply3/1
  Matrix Multiply6/1 -> M/1
  theta/1 -> arm to body/1(theta)

== system HighLevelLowLevel_SITLA 2/Tilt Rotor Simulator/Vehicle dynamics/Arm 3/Prop Froces and moment1 ==
  note: T = Ctx w^2
      | Q = Cd x w^2
  Cd : Inport
  Ct : Inport  Port=2
  omega : Inport  Port=3
  Product{,1..3} (4 alike) : Product
  F : Outport
  M : Outport  Port=2
  wires:
  omega/1 -> Product3/1, Product2/2, Product1/2, Product/2
  Ct/1 -> Product2/1
  Product2/1 -> Product3/2
  Product3/1 -> F/1
  Product/1 -> Product1/1
  Product1/1 -> M/1
  Cd/1 -> Product/1

== system HighLevelLowLevel_SITLA 2/Tilt Rotor Simulator/Vehicle dynamics/Arm 3/Subsystem2 ==
  In1 : Inport
  Derivative : Derivative
  Derivative1 : Derivative
  Transfer Fcn (with initial states)1 : simulink_extras/Additional Linear/Transfer Fcn (with initial states)  N=[153.5000]  D="[1  20.06  153.3]"  X0=0
  theta : Outport
  thetadot : Outport  Port=2
  thetadotdot : Outport  Port=3
  wires:
  Derivative/1 -> thetadot/1, Derivative1/1
  Transfer Fcn (with initial states)1/1 -> Derivative/1, theta/1
  Derivative1/1 -> thetadotdot/1
  In1/1 -> Transfer Fcn (with initial states)1/1

== system HighLevelLowLevel_SITLA 2/Tilt Rotor Simulator/Vehicle dynamics/Arm 3/Subsystem3 ==
  In1 : Inport
  Derivative2 : Derivative
  Derivative3 : Derivative
  Transfer Fcn (with initial states) : simulink_extras/Additional Linear/Transfer Fcn (with initial states)  N=[153.5000]  D="[1  20.06  153.3]"  X0=0
  phi : Outport
  phidot : Outport  Port=2
  phidotdot : Outport  Port=3
  wires:
  Derivative2/1 -> phidot/1, Derivative3/1
  Transfer Fcn (with initial states)/1 -> Derivative2/1, phi/1
  Derivative3/1 -> phidotdot/1
  In1/1 -> Transfer Fcn (with initial states)/1

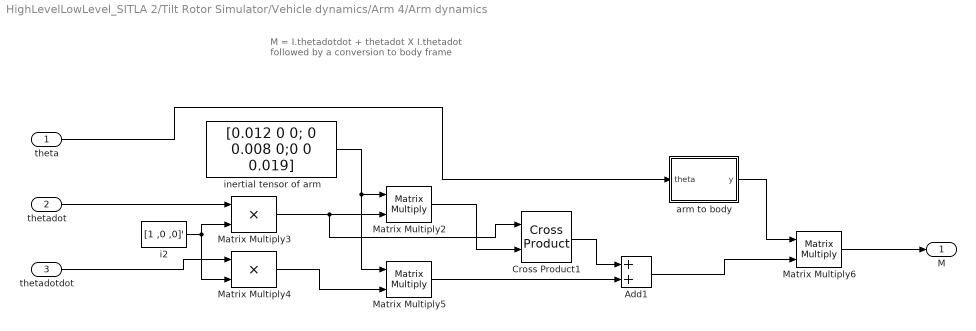
== system HighLevelLowLevel_SITLA 2/Tilt Rotor Simulator/Vehicle dynamics/Arm 4/Arm dynamics ==
  note: M = I.thetadotdot + thetadot X I.thetadot
      | followed by a conversion to body frame
  theta : Inport
  thetadot : Inport  Port=2
  thetadotdot : Inport  Port=3
  Add1 : Sum
  Cross Product1 : matrix_library/Cross Product
  Matrix Multiply2 : Product  Multiplication=Matrix(*)
  Matrix Multiply3 : Product
  Matrix Multiply4 : Product
  Matrix Multiply5 : Product  Multiplication=Matrix(*)
  Matrix Multiply6 : Product  Multiplication=Matrix(*)
  arm to body : MATLAB Function  TreatAsAtomicUnit=on
  i2 : Constant  Value=[1 ,0 ,0]'
  inertial tensor of arm : Constant  Value=[0.012 0 0; 0 0.008 0;0 0 0.019]
  M : Outport
  wires:
  Matrix Multiply3/1 -> Cross Product1/1, Matrix Multiply2/2
  inertial tensor of arm/1 -> Matrix Multiply5/1, Matrix Multiply2/1
  thetadotdot/1 -> Matrix Multiply4/1
  Matrix Multiply4/1 -> Matrix Multiply5/2
  Matrix Multiply5/1 -> Add1/2
  i2/1 -> Matrix Multiply4/2, Matrix Multiply3/2
  arm to body/1(y) -> Matrix Multiply6/1
  Matrix Multiply2/1 -> Cross Product1/2
  Cross Product1/1 -> Add1/1
  Add1/1 -> Matrix Multiply6/2
  thetadot/1 -> Matrix Multiply3/1
  Matrix Multiply6/1 -> M/1
  theta/1 -> arm to body/1(theta)

== system HighLevelLowLevel_SITLA 2/Tilt Rotor Simulator/Vehicle dynamics/Arm 4/Prop Froces and moment1 ==
  note: T = Ctx w^2
      | Q = Cd x w^2
  Cd : Inport
  Ct : Inport  Port=2
  omega : Inport  Port=3
  Product{,1..3} (4 alike) : Product
  F : Outport
  M : Outport  Port=2
  wires:
  omega/1 -> Product3/1, Product2/2, Product1/2, Product/2
  Ct/1 -> Product2/1
  Product2/1 -> Product3/2
  Product3/1 -> F/1
  Product/1 -> Product1/1
  Product1/1 -> M/1
  Cd/1 -> Product/1

== system HighLevelLowLevel_SITLA 2/Tilt Rotor Simulator/Vehicle dynamics/Arm 4/Subsystem2 ==
  In1 : Inport
  Derivative : Derivative
  Derivative1 : Derivative
  Transfer Fcn (with initial states)1 : simulink_extras/Additional Linear/Transfer Fcn (with initial states)  N=[153.5000]  D="[1  20.06  153.3]"  X0=0
  theta : Outport
  thetadot : Outport  Port=2
  thetadotdot : Outport  Port=3
  wires:
  Derivative/1 -> thetadot/1, Derivative1/1
  Transfer Fcn (with initial states)1/1 -> Derivative/1, theta/1
  Derivative1/1 -> thetadotdot/1
  In1/1 -> Transfer Fcn (with initial states)1/1

== system HighLevelLowLevel_SITLA 2/Tilt Rotor Simulator/Vehicle dynamics/Arm 4/Subsystem3 ==
  In1 : Inport
  Derivative2 : Derivative
  Derivative3 : Derivative
  Transfer Fcn (with initial states) : simulink_extras/Additional Linear/Transfer Fcn (with initial states)  N=[153.5000]  D="[1  20.06  153.3]"  X0=0
  phi : Outport
  phidot : Outport  Port=2
  phidotdot : Outport  Port=3
  wires:
  Derivative2/1 -> phidot/1, Derivative3/1
  Transfer Fcn (with initial states)/1 -> Derivative2/1, phi/1
  Derivative3/1 -> phidotdot/1
  In1/1 -> Transfer Fcn (with initial states)/1

== matlab function HighLevelLowLevel_SITLA 2/Tilt Rotor Simulator/Vehicle dynamics/Arm 3/prop to body1 ==
  data: theta input; phi input; y output
function y = fcn(theta, phi)

y = [sin(phi); -sin(theta)*cos(phi); cos(theta)*cos(phi)]; %derived in the literature

== matlab function HighLevelLowLevel_SITLA 2/Tilt Rotor Simulator/Vehicle dynamics/Arm 2/prop to body ==
  data: theta input; phi input; y output
function y = fcn(theta, phi)

y = [sin(phi); -sin(theta)*cos(phi); cos(theta)*cos(phi)]; %derived in the literature

== matlab function HighLevelLowLevel_SITLA 2/Tilt Rotor Simulator/Vehicle dynamics/Arm 4/Arm dynamics/arm to body ==
  data: theta input; y output
function y = fcn(theta)

theta = -theta; %negating because rotation is from arm to body frame, so angle of rotation will be opposite that of that arm

y = [1 0 0;
    0 cos(theta) -sin(theta);
    0 sin(theta) cos(theta)]; %a rotation about x axis

== matlab function HighLevelLowLevel_SITLA 2/Tilt Rotor Simulator/Vehicle dynamics/Arm 4/prop to body1 ==
  data: theta input; phi input; y output
function y = fcn(theta, phi)

y = [sin(phi); -sin(theta)*cos(phi); cos(theta)*cos(phi)]; %derived in the literature

== matlab function HighLevelLowLevel_SITLA 2/Tilt Rotor Simulator/Subsystem1/Subsystem/MATLAB Function10 ==
  data: u input; max_out parameter; min_out parameter; max_in parameter; y output; min_in parameter
function y = fcn(u, max_out, min_out, max_in, min_in)

y = (max_out - min_out) / (max_in - min_in) *(u - (min_in + max_in)/2) + (max_out + min_out)/2;

== matlab function HighLevelLowLevel_SITLA 2/Tilt Rotor Simulator/Subsystem1/Subsystem/MATLAB Function1 ==
  data: u input; max_out parameter; min_out parameter; max_in parameter; y output; min_in parameter
function y = fcn(u, max_out, min_out, max_in, min_in)

y = (max_out - min_out) / (max_in - min_in) *(u - (min_in + max_in)/2) + (max_out + min_out)/2;

== matlab function HighLevelLowLevel_SITLA 2/Tilt Rotor Simulator/Subsystem1/Subsystem/MATLAB Function11 ==
  data: u input; max_out parameter; min_out parameter; max_in parameter; y output; min_in parameter
function y = fcn(u, max_out, min_out, max_in, min_in)

y = (max_out - min_out) / (max_in - min_in) *(u - (min_in + max_in)/2) + (max_out + min_out)/2;

== matlab function HighLevelLowLevel_SITLA 2/Tilt Rotor Simulator/Vehicle dynamics/Arm 2/Arm dynamics/arm to body ==
  data: theta input; y output
function y = fcn(theta)

theta = -theta; %negating because rotation is from arm to body frame, so angle of rotation will be opposite that of that arm

y = [1 0 0;
    0 cos(theta) -sin(theta);
    0 sin(theta) cos(theta)]; %a rotation about x axis

== matlab function HighLevelLowLevel_SITLA 2/Tilt Rotor Simulator/Vehicle dynamics/Arm 1/prop to body1 ==
  data: theta input; phi input; y output
function y = fcn(theta, phi)

y = [sin(phi); -sin(theta)*cos(phi); cos(theta)*cos(phi)]; %derived in the literature

== matlab function HighLevelLowLevel_SITLA 2/Tilt Rotor Simulator/Subsystem1/Subsystem/MATLAB Function12 ==
  data: u input; max_out parameter; min_out parameter; max_in parameter; y output; min_in parameter
function y = fcn(u, max_out, min_out, max_in, min_in)

y = (max_out - min_out) / (max_in - min_in) *(u - (min_in + max_in)/2) + (max_out + min_out)/2;

== matlab function HighLevelLowLevel_SITLA 2/Tilt Rotor Simulator/Subsystem1/Subsystem/MATLAB Function9 ==
  data: u input; max_out parameter; min_out parameter; max_in parameter; y output; min_in parameter
function y = fcn(u, max_out, min_out, max_in, min_in)

y = (max_out - min_out) / (max_in - min_in) *(u - (min_in + max_in)/2) + (max_out + min_out)/2;

== matlab function HighLevelLowLevel_SITLA 2/Tilt Rotor Simulator/Simulated floor ==
  data: x input; F output; x1 parameter; x2 parameter; thickness parameter; E parameter; A parameter
function F   = wall(x, x1, x2, thickness, E, A)
    [d, direction] = point_to_line_segment_distance(x, x1, x2);
    if d <= thickness
        forceMagnitude = E * (thickness - d)/thickness * A;
        F = forceMagnitude * direction;
    else
        F = [0; 0; 0];
    end
end

function [d, direction] = point_to_line_segment_distance(x, a, b)
    ab = b - a; 
    ax = x(2:3) - a; 
    t = dot(ax, ab) / dot(ab, ab);
    t = max(0, min(1, t));
    closestPoint = a + t * ab;
    normal = [-ab(2); ab(1)];
    if dot(normal, ax) < 0
        normal = -normal;
    end
    direction = normal / norm(normal);
    direction = [0; direction];
    d = norm(x(2:3) - closestPoint);
end

== matlab function HighLevelLowLevel_SITLA 2/Tilt Rotor Simulator/Simulated Barrier ==
  data: x input; F output; x1 parameter; x2 parameter; thickness parameter; E parameter; A parameter
function F   = wall(x, x1, x2, thickness, E, A)
    [d, direction] = point_to_line_segment_distance(x, x1, x2);
    if d <= thickness
        forceMagnitude = E * (thickness - d)/thickness * A;
        F = forceMagnitude * direction;
    else
        F = [0; 0; 0];
    end
end

function [d, direction] = point_to_line_segment_distance(x, a, b)
    ab = b - a; 
    ax = x(1:2) - a; 
    t = dot(ax, ab) / dot(ab, ab);
    t = max(0, min(1, t));
    closestPoint = a + t * ab;
    normal = [-ab(2); ab(1)];
    if dot(normal, ax) < 0
        normal = -normal;
    end
    direction = normal / norm(normal);
    direction = [direction; 0];
    d = norm(x(1:2) - closestPoint);
end

== matlab function HighLevelLowLevel_SITLA 2/Tilt Rotor Simulator/Subsystem1/Subsystem/MATLAB Function6 ==
  data: u input; max_out parameter; min_out parameter; max_in parameter; y output; min_in parameter
function y = fcn(u, max_out, min_out, max_in, min_in)

y = (max_out - min_out) / (max_in - min_in) *(u - (min_in + max_in)/2) + (max_out + min_out)/2;

== matlab function HighLevelLowLevel_SITLA 2/Tilt Rotor Simulator/Subsystem1/Subsystem/MATLAB Function2 ==
  data: u input; max_out parameter; min_out parameter; max_in parameter; y output; min_in parameter
function y = fcn(u, max_out, min_out, max_in, min_in)

y = (max_out - min_out) / (max_in - min_in) *(u - (min_in + max_in)/2) + (max_out + min_out)/2;

== matlab function HighLevelLowLevel_SITLA 2/Tilt Rotor Simulator/Subsystem1/Subsystem/MATLAB Function3 ==
  data: u input; max_out parameter; min_out parameter; max_in parameter; y output; min_in parameter
function y = fcn(u, max_out, min_out, max_in, min_in)

y = (max_out - min_out) / (max_in - min_in) *(u - (min_in + max_in)/2) + (max_out + min_out)/2;

== matlab function HighLevelLowLevel_SITLA 2/Tilt Rotor Simulator/Subsystem1/Subsystem/MATLAB Function4 ==
  data: u input; max_out parameter; min_out parameter; max_in parameter; y output; min_in parameter
function y = fcn(u, max_out, min_out, max_in, min_in)

y = (max_out - min_out) / (max_in - min_in) *(u - (min_in + max_in)/2) + (max_out + min_out)/2;

== matlab function HighLevelLowLevel_SITLA 2/Tilt Rotor Simulator/Subsystem1/Subsystem/MATLAB Function5 ==
  data: u input; max_out parameter; min_out parameter; max_in parameter; y output; min_in parameter
function y = fcn(u, max_out, min_out, max_in, min_in)

y = (max_out - min_out) / (max_in - min_in) *(u - (min_in + max_in)/2) + (max_out + min_out)/2;

== matlab function HighLevelLowLevel_SITLA 2/Tilt Rotor Simulator/Subsystem1/Subsystem/MATLAB Function7 ==
  data: u input; max_out parameter; min_out parameter; max_in parameter; y output; min_in parameter
function y = fcn(u, max_out, min_out, max_in, min_in)

y = (max_out - min_out) / (max_in - min_in) *(u - (min_in + max_in)/2) + (max_out + min_out)/2;

== matlab function HighLevelLowLevel_SITLA 2/Tilt Rotor Simulator/Subsystem1/Subsystem/MATLAB Function8 ==
  data: u input; max_out parameter; min_out parameter; max_in parameter; y output; min_in parameter
function y = fcn(u, max_out, min_out, max_in, min_in)

y = (max_out - min_out) / (max_in - min_in) *(u - (min_in + max_in)/2) + (max_out + min_out)/2;

== matlab function HighLevelLowLevel_SITLA 2/Tilt Rotor Simulator/Vehicle dynamics/Arm 3/Arm dynamics/arm to body ==
  data: theta input; y output
function y = fcn(theta)

theta = -theta; %negating because rotation is from arm to body frame, so angle of rotation will be opposite that of that arm

y = [1 0 0;
    0 cos(theta) -sin(theta);
    0 sin(theta) cos(theta)]; %a rotation about x axis

== matlab function HighLevelLowLevel_SITLA 2/Tilt Rotor Simulator/Vehicle dynamics/Arm 1/Arm dynamics/arm to body ==
  data: theta input; y output
function y = fcn(theta)

theta = -theta; %negating because rotation is from arm to body frame, so angle of rotation will be opposite that of that arm

y = [1 0 0;
    0 cos(theta) -sin(theta);
    0 sin(theta) cos(theta)]; %a rotation about x axis
